simulink model "HeBon_function"  (R2020b)
settings: Solver=ode4  StartTime=0.0  StopTime=800  FixedStep=5  RelTol=1e-3
libraries: fuzblock x1
settings Model: Creator=Long  LastModifiedBy=Long
settings SolverCC: AlgebraicLoopSolver=LineSearch

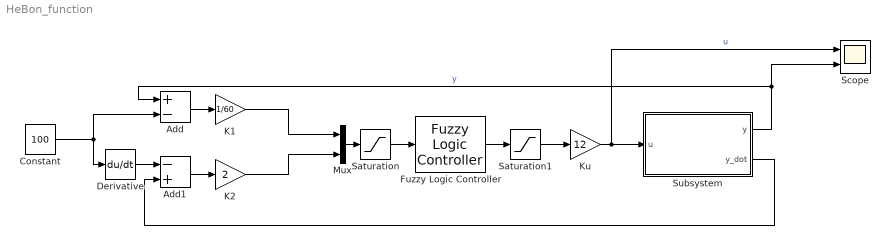
== system HeBon_function ==
  Add : Sum  Inputs=+-
  Add1 : Sum  Inputs=-+
  Constant : Constant  Value=100
  Derivative : Derivative
  Fuzzy Logic Controller : fuzblock/Fuzzy Logic  Controller  FIS='HeBon_FuzzyController.fis'  OutputSampleNumber=101  DataType=double  FuzzifiedInputs=off  RuleFiringStrengths=off  RuleOutputs=off  AggregatedOutputs=off  SimulateUsing=Interpreted execution  OutOfRangeInputValueMessage=warning  NoRuleFiredMessage=warning  EmptyOutputFuzzySetMessage=warning
  K1 : Gain  Gain=1/60
  K2 : Gain  Gain=2
  Ku : Gain  Gain=12
  Mux : Mux  Inputs=2
  Saturation : Saturate  UpperLimit=1  LowerLimit=-1
  Saturation1 : Saturate  UpperLimit=12  LowerLimit=0
  Scope : Scope  NumInputPorts=2
  Subsystem : Subsystem  mask{y0=0}
  wires:
  Subsystem/1(y) -> Scope/2, Add/1  "y"
  Constant/1 -> Add/2, Derivative/1
  K1/1 -> Mux/1
  K2/1 -> Mux/2
  Mux/1 -> Saturation/1
  Fuzzy Logic Controller/1 -> Saturation1/1
  Ku/1 -> Scope/1, Subsystem/1(u)  "u"
  Subsystem/2(y_dot) -> Add1/2
  Derivative/1 -> Add1/1
  Add/1 -> K1/1
  Add1/1 -> K2/1
  Saturation/1 -> Fuzzy Logic Controller/1
  Saturation1/1 -> Ku/1

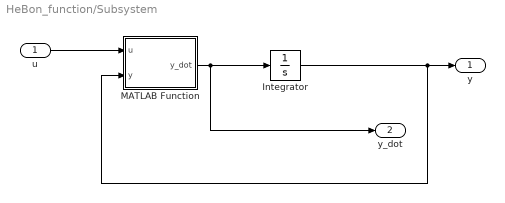
== system HeBon_function/Subsystem ==
  u : Inport
  Integrator : Integrator  InitialCondition=y0
  MATLAB Function : MATLAB Function  TreatAsAtomicUnit=on
  y : Outport
  y_dot : Outport  Port=2
  wires:
  MATLAB Function/1(y_dot) -> y_dot/1, Integrator/1
  u/1 -> MATLAB Function/1(u)
  Integrator/1 -> MATLAB Function/2(y), y/1

== matlab function HeBon_function/Subsystem/MATLAB Function ==
  data: u input; y_dot output; y input
function y_dot= fcn(u,y)
K = 140;
A = 314;
C = 0.9;
g = 9.81;
y_dot = (K*u-C*sqrt(2*g*y))/A;
